simulink model "PPC_P1_observer"  (R2019a)
settings: Solver=VariableStepAuto  StartTime=0.0  StopTime=20  RelTol=1e-3
settings Model: Creator=morga  LastModifiedBy=morga

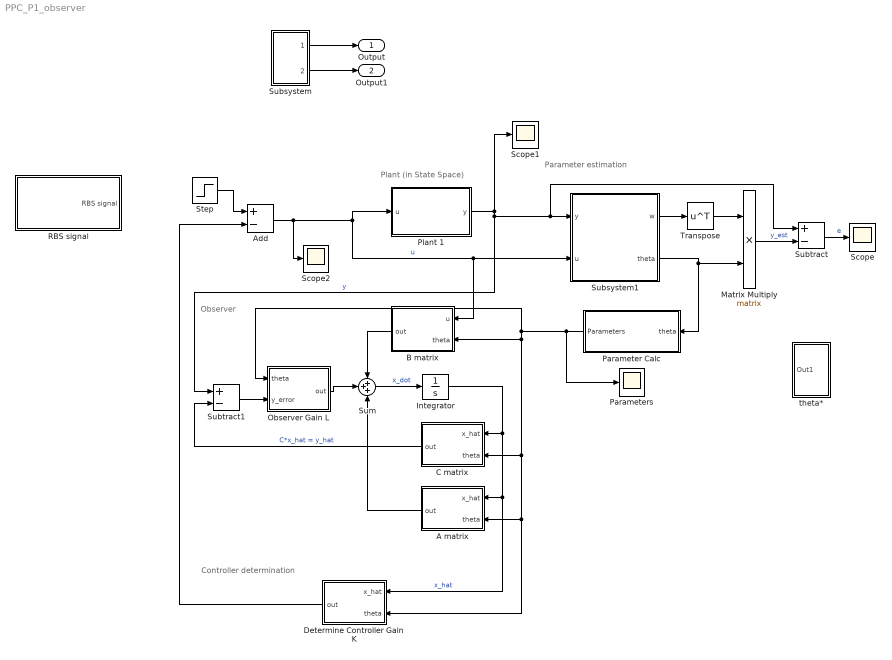
== system PPC_P1_observer ==
  note: Observer
  note: Parameter estimation
  note: Plant (in State Space)
  note: Controller determination
  A matrix : MATLAB Function  TreatAsAtomicUnit=on
  Add : Sum  Inputs=+-
  B matrix : MATLAB Function  TreatAsAtomicUnit=on
  C matrix : MATLAB Function  TreatAsAtomicUnit=on
  Determine Controller Gain K : MATLAB Function  TreatAsAtomicUnit=on
  Integrator : Integrator
  Matrix Multiply : Product  Multiplication=Matrix(*)
  Observer Gain L : MATLAB Function  TreatAsAtomicUnit=on
  Parameter Calc : Subsystem
  Parameters : Scope
  Plant 1 : Subsystem
  RBS signal : Subsystem
  Scope : Scope
  Scope1 : Scope
  Scope2 : Scope
  Step : Step  SampleTime=0
  Subsystem : Subsystem
  Subsystem1 : Subsystem
  Subtract : Sum  Inputs=+-
  Subtract1 : Sum  Inputs=+-
  Sum : Sum  Inputs=+++
  Transpose : Math  Operator=transpose  SaturateOnIntegerOverflow=on
  theta* : Subsystem
  Output : Outport
  Output1 : Outport  Port=2
  wires:
  Subsystem/1(Output) -> Output/1
  Subsystem/2(Output1) -> Output1/1
  Subsystem1/2(theta) -> Parameter Calc/1(theta), Matrix Multiply/2
  Plant 1/1(y) -> Scope1/1, Subtract1/1, Subtract/1, Subsystem1/1(y)  "y"
  Add/1 -> Scope2/1, Plant 1/1(u), B matrix/1(u), Subsystem1/2(u)  "u"
  Subsystem1/1(w) -> Transpose/1
  Transpose/1 -> Matrix Multiply/1
  Matrix Multiply/1 -> Subtract/2  "y_est"
  Subtract/1 -> Scope/1  "e"
  Determine Controller Gain K/1(out) -> Add/2
  Step/1 -> Add/1
  Parameter Calc/1(Parameters) -> Parameters/1, Determine Controller Gain K/2(theta), A matrix/2(theta), C matrix/2(theta), B matrix/2(theta), Observer Gain L/1(theta)
  Subtract1/1 -> Observer Gain L/2(y_error)
  Observer Gain L/1(out) -> Sum/2
  B matrix/1(out) -> Sum/1
  Sum/1 -> Integrator/1  "x_dot"
  Integrator/1 -> Determine Controller Gain K/1(x_hat), A matrix/1(x_hat), C matrix/1(x_hat)  "x_hat"
  C matrix/1(out) -> Subtract1/2  "C*x_hat = y_hat"
  A matrix/1(out) -> Sum/3

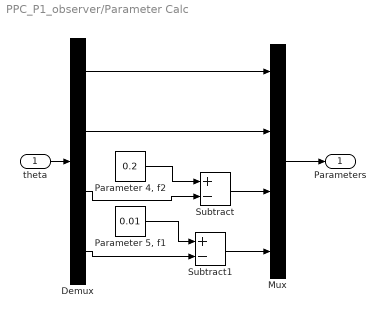
== system PPC_P1_observer/Parameter Calc ==
  theta : Inport
  Demux : Demux
  Mux : Mux
  "Parameter 4, f2" : Constant  Value=0.2
  "Parameter 5, f1" : Constant  Value=0.01
  Subtract : Sum  Inputs=+-
  Subtract1 : Sum  Inputs=+-
  Parameters : Outport
  wires:
  theta/1 -> Demux/1
  Demux/1 -> Mux/1
  Demux/2 -> Mux/2
  "Parameter 4, f2"/1 -> Subtract/1
  "Parameter 5, f1"/1 -> Subtract1/1
  Demux/4 -> Subtract1/2
  Demux/3 -> Subtract/2
  Subtract/1 -> Mux/3
  Subtract1/1 -> Mux/4
  Mux/1 -> Parameters/1

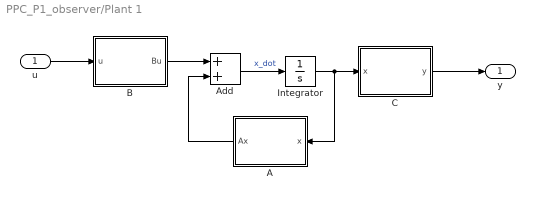
== system PPC_P1_observer/Plant 1 ==
  u : Inport  PortDimensions=1
  A : MATLAB Function  TreatAsAtomicUnit=on
  Add : Sum
  B : MATLAB Function  TreatAsAtomicUnit=on
  C : MATLAB Function  TreatAsAtomicUnit=on
  Integrator : Integrator  InitialCondition=[0 0]
  y : Outport
  wires:
  B/1(Bu) -> Add/1
  A/1(Ax) -> Add/2
  Add/1 -> Integrator/1  "x_dot"
  Integrator/1 -> A/1(x), C/1(x)
  C/1(y) -> y/1
  u/1 -> B/1(u)

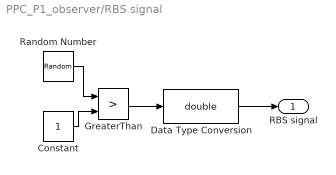
== system PPC_P1_observer/RBS signal ==
  Constant : Constant
  Data Type Conversion : DataTypeConversion  OutDataTypeStr=double
  GreaterThan : RelationalOperator  Operator=>  OutDataTypeStr=boolean  RndMeth=Simplest
  Random Number : RandomNumber  Mean=1  SampleTime=0.1
  RBS signal : Outport
  wires:
  Random Number/1 -> GreaterThan/1
  Data Type Conversion/1 -> RBS signal/1
  GreaterThan/1 -> Data Type Conversion/1
  Constant/1 -> GreaterThan/2

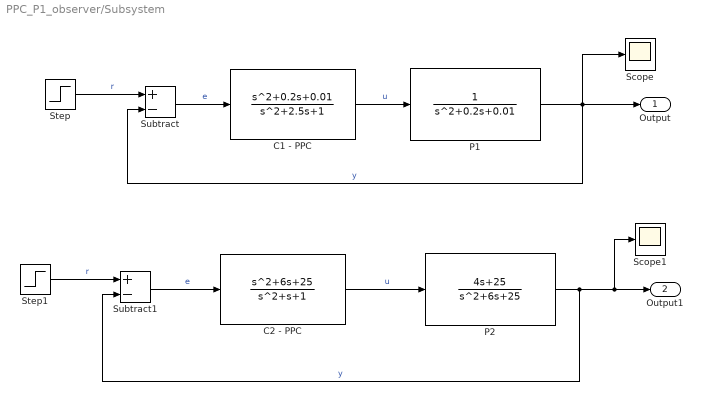
== system PPC_P1_observer/Subsystem ==
  C1 - PPC : TransferFcn  Numerator=[1 0.2 0.01]  Denominator=[1 2.5 1]
  C2 - PPC : TransferFcn  Numerator=[1 6 25]  Denominator=[1 1 1]
  P1 : TransferFcn  Denominator=[1 0.2 0.01]
  P2 : TransferFcn  Numerator=[4 25]  Denominator=[1 6 25]
  Scope : Scope
  Scope1 : Scope
  Step : Step  SampleTime=0
  Step1 : Step  SampleTime=0
  Subtract : Sum  Inputs=+-
  Subtract1 : Sum  Inputs=+-
  Output : Outport
  Output1 : Outport  Port=2
  wires:
  C1 - PPC/1 -> P1/1  "u"
  P1/1 -> Output/1, Scope/1, Subtract/2  "y"
  P2/1 -> Output1/1, Scope1/1, Subtract1/2  "y"
  Step/1 -> Subtract/1  "r"
  C2 - PPC/1 -> P2/1  "u"
  Subtract/1 -> C1 - PPC/1  "e"
  Subtract1/1 -> C2 - PPC/1  "e"
  Step1/1 -> Subtract1/1  "r"

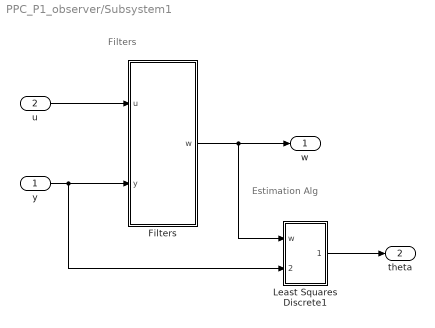
== system PPC_P1_observer/Subsystem1 ==
  note: Estimation Alg
  note: Filters
  y : Inport
  u : Inport  Port=2
  Filters : Subsystem
  Least Squares Discrete1 : Subsystem
  w : Outport
  theta : Outport  Port=2
  wires:
  u/1 -> Filters/1(u)
  y/1 -> Least Squares Discrete1/2(Y_p), Filters/2(y)
  Filters/1(w) -> w/1, Least Squares Discrete1/1(w)
  Least Squares Discrete1/1(theta) -> theta/1

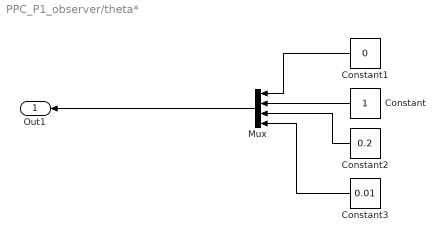
== system PPC_P1_observer/theta* ==
  Constant : Constant
  Constant1 : Constant  Value=0
  Constant2 : Constant  Value=0.2
  Constant3 : Constant  Value=0.01
  Mux : Mux
  Out1 : Outport
  wires:
  Constant/1 -> Mux/2
  Constant3/1 -> Mux/4
  Constant2/1 -> Mux/3
  Constant1/1 -> Mux/1
  Mux/1 -> Out1/1

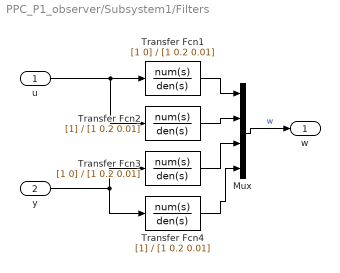
== system PPC_P1_observer/Subsystem1/Filters ==
  u : Inport  PortDimensions=1
  y : Inport  Port=2
  Mux : Mux
  Transfer Fcn1 : TransferFcn  Numerator=[1 0]  Denominator=[1 0.2 0.01]
  Transfer Fcn2 : TransferFcn  Denominator=[1 0.2 0.01]
  Transfer Fcn3 : TransferFcn  Numerator=[1 0]  Denominator=[1 0.2 0.01]
  Transfer Fcn4 : TransferFcn  Denominator=[1 0.2 0.01]
  w : Outport
  wires:
  Transfer Fcn2/1 -> Mux/2
  u/1 -> Transfer Fcn2/1, Transfer Fcn1/1
  Transfer Fcn3/1 -> Mux/3
  y/1 -> Transfer Fcn3/1, Transfer Fcn4/1
  Transfer Fcn1/1 -> Mux/1
  Mux/1 -> w/1  "w"
  Transfer Fcn4/1 -> Mux/4

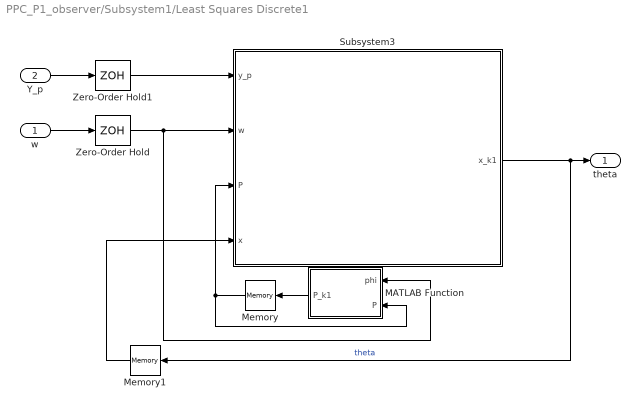
== system PPC_P1_observer/Subsystem1/Least Squares Discrete1 ==
  w : Inport
  Y_p : Inport  Port=2
  MATLAB Function : MATLAB Function  TreatAsAtomicUnit=on
  Memory : Memory  InitialCondition=100000*eye(4)
  Memory1 : Memory  InitialCondition=[0 0 0 0]
  Subsystem3 : Subsystem
  Zero-Order Hold : ZeroOrderHold  SampleTime=0.001
  Zero-Order Hold1 : ZeroOrderHold  SampleTime=0.001
  theta : Outport
  wires:
  Subsystem3/1(x_k1) -> Memory1/1, theta/1  "theta"
  MATLAB Function/1(P_k1) -> Memory/1
  w/1 -> Zero-Order Hold/1
  Zero-Order Hold1/1 -> Subsystem3/1(y_p)
  Memory/1 -> Subsystem3/3(P), MATLAB Function/2(P)
  Zero-Order Hold/1 -> MATLAB Function/1(phi), Subsystem3/2(w)
  Y_p/1 -> Zero-Order Hold1/1
  Memory1/1 -> Subsystem3/4(x)

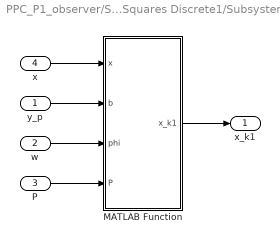
== system PPC_P1_observer/Subsystem1/Least Squares Discrete1/Subsystem3 ==
  y_p : Inport
  w : Inport  Port=2
  P : Inport  Port=3
  x : Inport  Port=4
  MATLAB Function : MATLAB Function  TreatAsAtomicUnit=on
  x_k1 : Outport
  wires:
  MATLAB Function/1(x_k1) -> x_k1/1
  y_p/1 -> MATLAB Function/2(b)
  P/1 -> MATLAB Function/4(P)
  w/1 -> MATLAB Function/3(phi)
  x/1 -> MATLAB Function/1(x)

== matlab function PPC_P1_observer/Subsystem1/Least Squares Discrete1/MATLAB Function ==
  data: phi input; P_k1 output; P input
function P_k1 = fcn(phi,P)
alpha = 1;
lambda = 1;

P_k1 = 1/alpha*P - (lambda*lambda*P*phi*phi'*P)/(1+lambda*phi'*P*phi);

== matlab function PPC_P1_observer/Determine Controller Gain K ==
  data: x_hat input; theta input; out output
function out = fcn(x_hat,theta)
% theta = estimations of parameters
% Goal of this function is to construct the estimated plant in terms of
% state space - A, B, C - and then determine the K controller that is
% appropriate to achieve desired pole placement (PPC control)
a0 = theta(4); a1 = theta(3); %values of A in CCF
p1 = -1; p2 = -1; % desired pole values
alpha = [-(p1+p2) p1*p2];

K = [alpha(2)-a0 alpha(1)-a1];
out = K*x_hat;

== matlab function PPC_P1_observer/Plant 1/A ==
  data: x input; Ax output
function Ax = fcn(x)
A = [0 1; -0.01 -0.2];
Ax = A*x;

== matlab function PPC_P1_observer/Plant 1/B ==
  data: u input; Bu output
function Bu = fcn(u)
B = [0 1]';
Bu = B*u;

== matlab function PPC_P1_observer/Plant 1/C ==
  data: x input; y output
function y = fcn(x)
C = [1 0];
y = C*x;

== matlab function PPC_P1_observer/Observer Gain L ==
  data: theta input; y_error input; out output
function out = fcn(theta,y_error)

a0 = theta(4); a1 = theta(3); %values of A in CCF
p1 = -10; p2 = -10; % desired pole values
alpha = [-(p1+p2) p1*p2];

L = [alpha(2)-a0 alpha(1)-a1];

out = L*y_error;

== matlab function PPC_P1_observer/Subsystem1/Least Squares Discrete1/Subsystem3/MATLAB Function ==
  data: x input; x_k1 output; b input; phi input; P input
function x_k1 = fcn(x,b,phi,P)
lambda = 1; 
% X_k1 = theta_k+1
% b = y(t)

x_k1 = x - (lambda*P*phi*(phi'*x-b))/(1+lambda*phi'*P*phi);

== matlab function PPC_P1_observer/B matrix ==
  data: u input; theta input; out output
function out = fcn(u, theta)

B = [0; 1];
out = B*u;

== matlab function PPC_P1_observer/C matrix ==
  data: x_hat input; theta input; out output
function out = fcn(x_hat, theta)
% theta = estimations of parameters

C = [theta(2) theta(1)];
out = C*x_hat;

== matlab function PPC_P1_observer/A matrix ==
  data: x_hat input; theta input; out output
function out = fcn(x_hat, theta)
a0 = theta(4); a1 = theta(3); %values of A in CCF 
A = [0 1; -a0 -a1];
out = A*x_hat;
